simulink model "test_com_AdaptiveTireModel"  (R2017a)
settings: Solver=FixedStepDiscrete  StartTime=450  StopTime=650  RelTol=1e-3
undefined symbols (not defined in the file or in its folder): AxleFrontX, AxleRearX, GearRatio, TireRDyn, TrackAngleFront, TrackWidthFront, TrackWidthRear
settings Model: DataDictionary=controller_dict.sldd  Creator=rieth  LastModifiedBy=rieth
settings DataIOCC: ExternalInput=VD_SteeringAngle_Value, VD_V2O_SpeedLongitudinal, VD_V2O_SpeedLateral, PT_Motor_MotorSpeed_FL, PT_Motor_MotorSpeed_FR, PT_Motor_MotorSpeed_RL, PT_Motor_MotorSpeed_RR, VD_Gyro_Front_Accel_X, VD_Gyro_Front_Accel_Y, VD_Gyro_Front_Accel_Z, VD_Gyro_Front_ARate_X, VD_Gyro_Front_ARate_Y, VD_Gyro_Front_ARate_Z, VD_Gyro_Front_Comp_X, VD_Gyro_Front_Comp_Y, VD_Gyro_Front_Comp_Z, VD_Gyro_Front_Temp, VD_Gyro_Rear_Accel_X, VD_Gyro_Rear_Accel_Y, VD_Gyro_Rear_Accel_Z, VD_Gyro_Rear_ARate_X, VD_Gyro_Rear_ARate_Y,VD_Gyro_Rear_ARate_Z, VD_Gyro_Rear_Comp_X, VD_Gyro_Rear_Comp_Y, VD_Gyro_Rear_Comp_Z, VD_Gyro_Rear_Temp, PT_TorqueCurrent_FL, PT_TorqueCurrent_FR, PT_TorqueCurrent_RL, PT_TorqueCurrent_RR,VD_Suspension_Hall_FL,VD_Suspension_Hall_FR,VD_Suspension_Hall_RL,VD_Suspension_Hall_RR  LoadExternalInput=on
settings OptimizationCC: UseDivisionForNetSlopeComputation=on

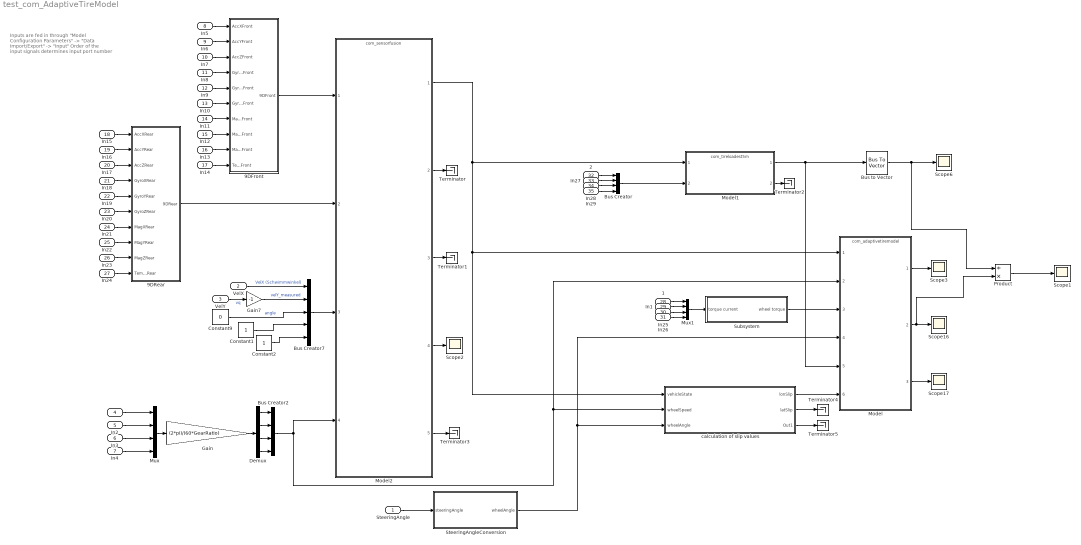
== system test_com_AdaptiveTireModel ==
  note: Inputs are fed in through "Model Configuration Parameters" ->
      | "Data Import/Export" -> "Input"
      | Order of the input signals determines input port number
  SteeringAngle : Inport  OutDataTypeStr=single  Interpolate=off
  VelX : Inport  Port=2  OutDataTypeStr=single
  VelY : Inport  Port=3  OutDataTypeStr=single
  " " : Inport  Port=4  OutDataTypeStr=single
  In2 : Inport  Port=5  OutDataTypeStr=single
  In3 : Inport  Port=6  OutDataTypeStr=single
  In4 : Inport  Port=7  OutDataTypeStr=single
  In5 : Inport  Port=8
  In6 : Inport  Port=9
  In7 : Inport  Port=10
  In8 : Inport  Port=11
  In9 : Inport  Port=12
  In10 : Inport  Port=13
  In11 : Inport  Port=14
  In12 : Inport  Port=15
  In13 : Inport  Port=16
  In14 : Inport  Port=17
  In15 : Inport  Port=18
  In16 : Inport  Port=19
  In17 : Inport  Port=20
  In18 : Inport  Port=21
  In19 : Inport  Port=22
  In20 : Inport  Port=23
  In21 : Inport  Port=24
  In22 : Inport  Port=25
  In23 : Inport  Port=26
  In24 : Inport  Port=27
  " 1" : Inport  Port=28  OutDataTypeStr=single
  In1 : Inport  Port=29  OutDataTypeStr=single
  In25 : Inport  Port=30  OutDataTypeStr=single
  In26 : Inport  Port=31  OutDataTypeStr=single
  " 2" : Inport  Port=32  OutDataTypeStr=single
  In27 : Inport  Port=33  OutDataTypeStr=single
  In28 : Inport  Port=34  OutDataTypeStr=single
  In29 : Inport  Port=35  OutDataTypeStr=single
  9DFront : Subsystem
  9DRear : Subsystem
  Bus Creator : BusCreator  Inputs=4  OutDataTypeStr=Bus: control_LinPot
  Bus Creator2 : BusCreator  Inputs=4  OutDataTypeStr=Bus: control_WheelSpeed
      settings: InheritFromInputs=off
  Bus Creator7 : BusCreator  Inputs=5  OutDataTypeStr=Bus: control_velocity
      settings: InheritFromInputs=off
  Bus to Vector : BusToVector
  Constant1 : Constant  OutDataTypeStr=Inherit: Inherit via back propagation
  Constant2 : Constant  OutDataTypeStr=Inherit: Inherit via back propagation
  Constant9 : Constant  Value=0  OutDataTypeStr=Inherit: Inherit via back propagation
  Demux : Demux
  Gain : Gain  Gain=(2*pi)/(60*GearRatio)
  Gain7 : Gain  Gain=-1
  Model : ModelReference  ModelNameDialog=com_adaptivetiremodel.slx  SimulationMode=Normal  ModelReferenceVersion=1.201
  Model1 : ModelReference  ModelNameDialog=com_tireloadest5m.slx  SimulationMode=Normal  ModelReferenceVersion=1.119
  Model2 : ModelReference  ModelNameDialog=com_sensorfusion.slx  SimulationMode=Normal  ModelReferenceVersion=1.1509
  Mux : Mux
  Mux1 : Mux
  Product : Product  Inputs=/*
  Scope{1..3,6,16..17} (6 alike) : Scope
  SteeringAngleConversion : Subsystem
  Subsystem : Subsystem
  Terminator{,1..5} (6 alike) : Terminator
  calculation of slip values : Subsystem
  wires:
  Model2/1 -> Model1/1, calculation of slip values/1(vehicleState), Model/1
  Model2/2 -> Terminator/1
  Model2/3 -> Terminator1/1
  Model1/1 -> Model/5, Bus to Vector/1
  Model/1 -> Scope3/1
  In23/1 -> 9DRear/9(MagZRear)
  In18/1 -> 9DRear/4(GyroXRear)
  In26/1 -> Mux1/4
  " 1"/1 -> Mux1/1
  Demux/3 -> Bus Creator2/3
  VelY/1 -> Gain7/1  "vq"
  Bus Creator7/1 -> Model2/3
  SteeringAngle/1 -> SteeringAngleConversion/1("steeringAngle ")
  In10/1 -> 9DFront/6(GyroZFront)
  VelX/1 -> Bus Creator7/1  "VelX (Schwimmwinkel)"
  Mux/1 -> Gain/1
  Subsystem/1(wheel torque) -> Model/3
  In1/1 -> Mux1/2
  In20/1 -> 9DRear/6(GyroZRear)
  Model/3 -> Scope17/1
  In16/1 -> 9DRear/2(AccYRear)
  In13/1 -> 9DFront/9(MagZFront)
  In12/1 -> 9DFront/8(MagYFront)
  In24/1 -> 9DRear/10(Temp9DRear)
  " "/1 -> Mux/1
  Demux/2 -> Bus Creator2/2
  Bus Creator2/1 -> Model2/4, Model/2, calculation of slip values/2(wheelSpeed)
  Gain7/1 -> Bus Creator7/2  "velY_measured"
  Constant9/1 -> Bus Creator7/3  "angle"
  Mux1/1 -> Subsystem/1(torque current)
  In15/1 -> 9DRear/1(AccXRear)
  In19/1 -> 9DRear/5(GyroYRear)
  In4/1 -> Mux/4
  In8/1 -> 9DFront/4(GyroXFront)
  In6/1 -> 9DFront/2(AccYFront)
  In2/1 -> Mux/2
  In5/1 -> 9DFront/1(AccXFront)
  In7/1 -> 9DFront/3(AccZFront)
  In14/1 -> 9DFront/10(Temp9DFront)
  Gain/1 -> Demux/1
  In17/1 -> 9DRear/3(AccZRear)
  In21/1 -> 9DRear/7(MagXRear)
  Demux/4 -> Bus Creator2/4
  In3/1 -> Mux/3
  In11/1 -> 9DFront/7(MagXFront)
  In25/1 -> Mux1/3
  In9/1 -> 9DFront/5(GyroYFront)
  Demux/1 -> Bus Creator2/1
  9DFront/1(9DFront) -> Model2/1
  Model/2 -> Product/2, Scope16/1
  9DRear/1(9DRear) -> Model2/2
  In22/1 -> 9DRear/8(MagYRear)
  Model2/5 -> Terminator3/1
  Model2/4 -> Scope2/1
  In28/1 -> Bus Creator/3
  In27/1 -> Bus Creator/2
  " 2"/1 -> Bus Creator/1
  In29/1 -> Bus Creator/4
  Bus Creator/1 -> Model1/2
  Model1/2 -> Terminator2/1
  Constant1/1 -> Bus Creator7/4
  Constant2/1 -> Bus Creator7/5
  Bus to Vector/1 -> Product/1, Scope6/1
  Product/1 -> Scope1/1
  calculation of slip values/2(latSlip) -> Terminator4/1
  calculation of slip values/1(lonSlip) -> Model/6
  calculation of slip values/3(Out1) -> Terminator5/1
  SteeringAngleConversion/1(wheelAngle) -> Model/4, calculation of slip values/3(wheelAngle)

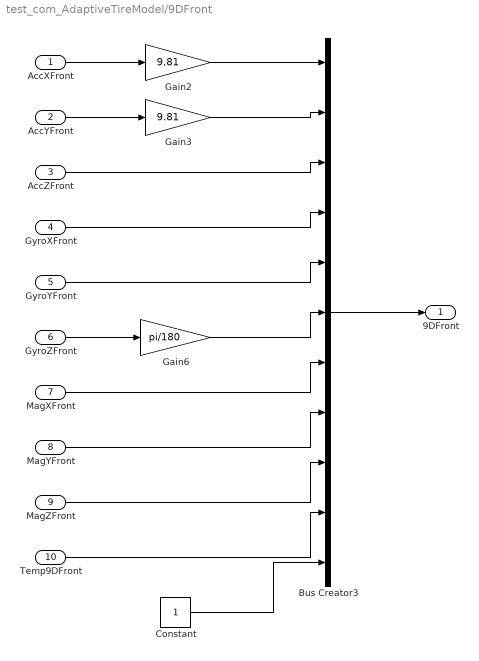
== system test_com_AdaptiveTireModel/9DFront ==
  AccXFront : Inport
  AccYFront : Inport  Port=2
  AccZFront : Inport  Port=3
  GyroXFront : Inport  Port=4
  GyroYFront : Inport  Port=5
  GyroZFront : Inport  Port=6
  MagXFront : Inport  Port=7
  MagYFront : Inport  Port=8
  MagZFront : Inport  Port=9
  Temp9DFront : Inport  Port=10
  Bus Creator3 : BusCreator  Inputs=11  OutDataTypeStr=Bus: control_9D_Full_float
      settings: InheritFromInputs=off
  Constant : Constant  OutDataTypeStr=Inherit: Inherit via back propagation
  Gain2 : Gain  Gain=9.81
  Gain3 : Gain  Gain=9.81
  Gain6 : Gain  Gain=pi/180
  9DFront : Outport
  wires:
  AccXFront/1 -> Gain2/1
  Temp9DFront/1 -> Bus Creator3/10
  GyroZFront/1 -> Gain6/1
  AccZFront/1 -> Bus Creator3/3
  AccYFront/1 -> Gain3/1
  GyroYFront/1 -> Bus Creator3/5
  MagZFront/1 -> Bus Creator3/9
  Gain2/1 -> Bus Creator3/1
  Bus Creator3/1 -> 9DFront/1
  MagYFront/1 -> Bus Creator3/8
  MagXFront/1 -> Bus Creator3/7
  Gain6/1 -> Bus Creator3/6
  GyroXFront/1 -> Bus Creator3/4
  Gain3/1 -> Bus Creator3/2
  Constant/1 -> Bus Creator3/11

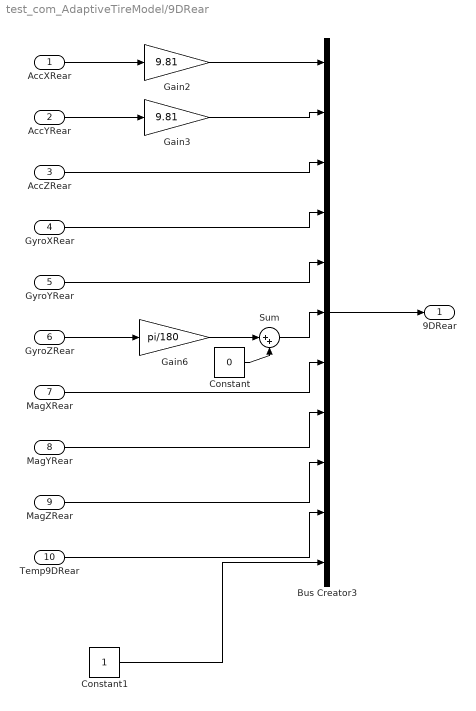
== system test_com_AdaptiveTireModel/9DRear ==
  AccXRear : Inport
  AccYRear : Inport  Port=2
  AccZRear : Inport  Port=3
  GyroXRear : Inport  Port=4
  GyroYRear : Inport  Port=5
  GyroZRear : Inport  Port=6
  MagXRear : Inport  Port=7
  MagYRear : Inport  Port=8
  MagZRear : Inport  Port=9
  Temp9DRear : Inport  Port=10
  Bus Creator3 : BusCreator  Inputs=11  OutDataTypeStr=Bus: control_9D_Full_float
      settings: InheritFromInputs=off
  Constant : Constant  Value=0  OutDataTypeStr=single
  Constant1 : Constant  OutDataTypeStr=Inherit: Inherit via back propagation
  Gain2 : Gain  Gain=9.81
  Gain3 : Gain  Gain=9.81
  Gain6 : Gain  Gain=pi/180
  Sum : Sum  Inputs=|++
  9DRear : Outport
  wires:
  GyroXRear/1 -> Bus Creator3/4
  Gain6/1 -> Sum/1
  MagXRear/1 -> Bus Creator3/7
  MagYRear/1 -> Bus Creator3/8
  Bus Creator3/1 -> 9DRear/1
  Gain3/1 -> Bus Creator3/2
  Gain2/1 -> Bus Creator3/1
  MagZRear/1 -> Bus Creator3/9
  GyroYRear/1 -> Bus Creator3/5
  AccYRear/1 -> Gain3/1
  AccZRear/1 -> Bus Creator3/3
  GyroZRear/1 -> Gain6/1
  Temp9DRear/1 -> Bus Creator3/10
  AccXRear/1 -> Gain2/1
  Sum/1 -> Bus Creator3/6
  Constant/1 -> Sum/2
  Constant1/1 -> Bus Creator3/11

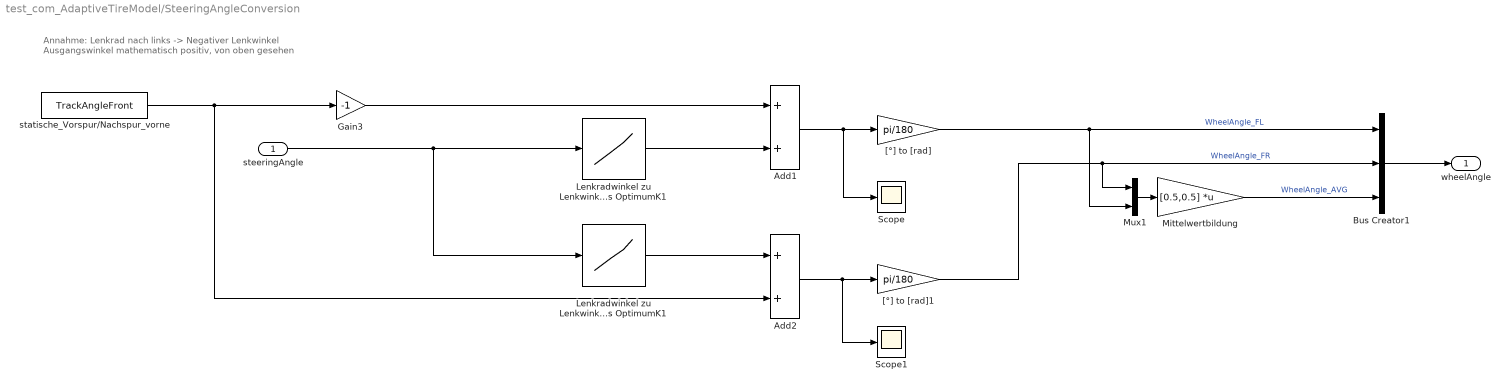
== system test_com_AdaptiveTireModel/SteeringAngleConversion ==
  note: Annahme: Lenkrad nach links -> Negativer Lenkwinkel
      | Ausgangswinkel mathematisch positiv, von oben gesehen
  "steeringAngle " : Inport  Unit=deg
  Add1 : Sum
  Add2 : Sum
  Bus Creator1 : BusCreator  Inputs=3  OutDataTypeStr=Bus: control_WheelAngle
  Gain3 : Gain  Gain=-1
  Lenkradwinkel zu Lenkwinkel_vl aus OptimumK1 : Lookup_n-D  NumberOfTableDimensions=1  BreakpointsForDimension1=|  Table=|  InternalRulePriority=Speed  RndMeth=Simplest  InputSameDT=on
      BreakpointsForDimension1=|
      | [-110
      | -99
      | -88
      | -77
      | -66
      | -55
      | -44
      | -33
      | -22
      | -11
      | 0
      | 11
      | 22
      | 33
      | 44
      | 55
      | 66
      | 77
      | 88
      | 99
      | 110]
      Table=|
      | [-31.406
      | -27.9
      | -24.526
      | -21.258
      | -18.075
      | -14.961
      | -11.902
      | -8.886
      | -5.903
      | -2.944
      | 0
      | 2.937
      | 5.874
      | 8.819
      | 11.78
      | 14.765
      | 17.781
      | 20.838
      | 23.945
      | 27.115
      | 30.358]
  Lenkradwinkel zu Lenkwinkel_vr aus OptimumK1 : Lookup_n-D  NumberOfTableDimensions=1  BreakpointsForDimension1=|  Table=|  InternalRulePriority=Speed  RndMeth=Simplest  InputSameDT=on
      BreakpointsForDimension1=|
      | [-110
      | -99
      | -88
      | -77
      | -66
      | -55
      | -44
      | -33
      | -22
      | -11
      | 0
      | 11
      | 22
      | 33
      | 44
      | 55
      | 66
      | 77
      | 88
      | 99
      | 110]
      Table=|
      | [-30.358
      | -27.115
      | -23.945
      | -20.838
      | -17.781
      | -14.765
      | -11.78
      | -8.819
      | -5.874
      | -2.937
      | 0
      | 2.944
      | 5.903
      | 8.886
      | 11.902
      | 14.961
      | 18.075
      | 21.258
      | 24.526
      | 27.9
      | 31.406]
  Mittelwertbildung : Gain  Gain=[0.5,0.5]  Multiplication=Matrix(K*u)
  Mux1 : Mux  Inputs=2
  Scope : Scope
  Scope1 : Scope
  "[°] to [rad]" : Gain  Gain=pi/180
  "[°] to [rad]1" : Gain  Gain=pi/180
  statische_Vorspur/Nachspur_vorne : Constant  Value=TrackAngleFront
  wheelAngle : Outport
  wires:
  Add2/1 -> Scope1/1, "[°] to [rad]1"/1
  statische_Vorspur/Nachspur_vorne/1 -> Add2/2, Gain3/1
  Lenkradwinkel zu Lenkwinkel_vl aus OptimumK1/1 -> Add1/2
  Lenkradwinkel zu Lenkwinkel_vr aus OptimumK1/1 -> Add2/1
  Gain3/1 -> Add1/1
  "steeringAngle "/1 -> Lenkradwinkel zu Lenkwinkel_vr aus OptimumK1/1, Lenkradwinkel zu Lenkwinkel_vl aus OptimumK1/1
  "[°] to [rad]"/1 -> Bus Creator1/1, Mux1/2  "WheelAngle_FL"
  Add1/1 -> "[°] to [rad]"/1, Scope/1
  "[°] to [rad]1"/1 -> Bus Creator1/2, Mux1/1  "WheelAngle_FR"
  Bus Creator1/1 -> wheelAngle/1
  Mux1/1 -> Mittelwertbildung/1
  Mittelwertbildung/1 -> Bus Creator1/3  "WheelAngle_AVG"

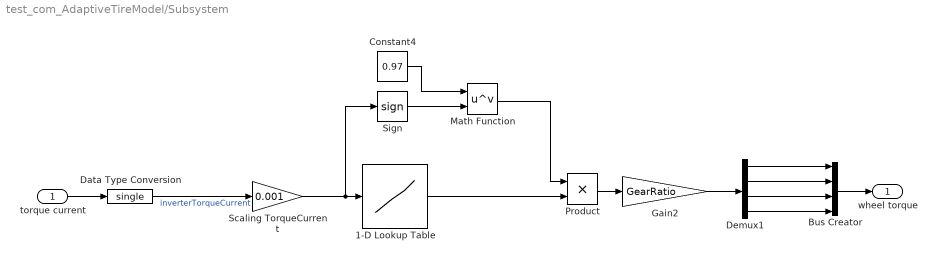
== system test_com_AdaptiveTireModel/Subsystem ==
  torque current : Inport
  1-D Lookup Table : Lookup_n-D  NumberOfTableDimensions=1  BreakpointsForDimension1=single([-98.31700100000001 -91.605003 -83.987999 -76.350998 -68.718002 -61.085999 -53.451 -45.814999 -38.173 -30.547001 -27.493999 -24.450001 -21.4 -18.35 -15.3 -12.26 -9.2110004 -6.1700001 -3.142 0 3.142 6.1700001 9.2110004 12.26 15.3 18.35 21.4 24.450001 27.493999 30.547001 38.173 45.814999 53.451 61.085999 68.718002 76.350998 83.987999 91.605003 98.31700100000001])  Table=single([-27.7 -26.7 -25.5 -24.1 -22.4 -20.5 -18.5 -16.2 -13.8 -11.2 -10.1 -9 -7.8 -6.7 -5.5 -4.4 -3.3 -2.1 -0.9 0 0.9 2.1 3.3 4.4 5.5 6.7 7.8 9 10.1 11.2 13.8 16.2 18.5 20.5 22.4 24.1 25.5 26.7 27.7])  InternalRulePriority=Speed  RndMeth=Simplest  InputSameDT=on
  Bus Creator : BusCreator  Inputs=4  OutDataTypeStr=Bus: control_WheelTorque
      settings: InheritFromInputs=off
  Constant4 : Constant  Value=0.97  OutDataTypeStr=Inherit: Inherit via back propagation
  Data Type Conversion : DataTypeConversion  OutDataTypeStr=single
  Demux1 : Demux
  Gain2 : Gain  Gain=GearRatio
  Math Function : Math  Operator=pow  OutputSignalType=real  SaturateOnIntegerOverflow=on
  Product : Product
  Scaling TorqueCurrent : Gain  Gain=0.001
  Sign : Signum
  wheel torque : Outport  OutDataTypeStr=Bus: control_WheelTorque
  wires:
  Bus Creator/1 -> wheel torque/1
  Gain2/1 -> Demux1/1
  Demux1/4 -> Bus Creator/4
  Demux1/1 -> Bus Creator/1
  Demux1/2 -> Bus Creator/2
  Demux1/3 -> Bus Creator/3
  torque current/1 -> Data Type Conversion/1
  Product/1 -> Gain2/1
  Math Function/1 -> Product/1
  1-D Lookup Table/1 -> Product/2
  Constant4/1 -> Math Function/1
  Data Type Conversion/1 -> Scaling TorqueCurrent/1  "inverterTorqueCurrent"
  Scaling TorqueCurrent/1 -> Sign/1, 1-D Lookup Table/1
  Sign/1 -> Math Function/2

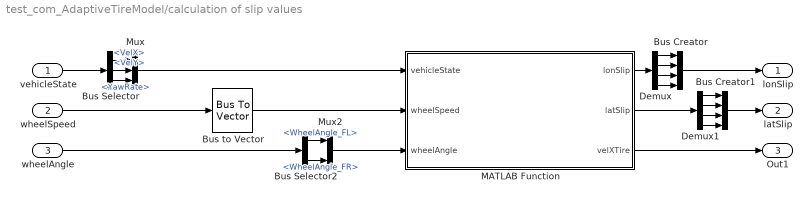
== system test_com_AdaptiveTireModel/calculation of slip values ==
  vehicleState : Inport  OutDataTypeStr=Bus: control_VehicleStateRB
  wheelSpeed : Inport  Port=2  OutDataTypeStr=Bus: control_WheelSpeed
  wheelAngle : Inport  Port=3  OutDataTypeStr=Bus: control_WheelAngle
  Bus Creator : BusCreator  Inputs=4  OutDataTypeStr=Bus: control_LonSlip
      settings: InheritFromInputs=off
  Bus Creator1 : BusCreator  Inputs=4  OutDataTypeStr=Bus: control_LatSlip
      settings: InheritFromInputs=off
  Bus Selector : BusSelector  OutputSignals=VelX,VelY,YawRate
  Bus Selector2 : BusSelector  OutputSignals=WheelAngle_FL,WheelAngle_FR
  Bus to Vector : BusToVector
  Demux : Demux
  Demux1 : Demux
  MATLAB Function : MATLAB Function  TreatAsAtomicUnit=on
  Mux : Mux  Inputs=3
  Mux2 : Mux  Inputs=2
  lonSlip : Outport
  latSlip : Outport  Port=2
  Out1 : Outport  Port=3
  wires:
  Bus Selector/3 -> Mux/3  "<YawRate>"
  Mux/1 -> MATLAB Function/1(vehicleState)
  vehicleState/1 -> Bus Selector/1
  Bus Selector/2 -> Mux/2  "<VelY>"
  Demux1/4 -> Bus Creator1/4
  wheelSpeed/1 -> Bus to Vector/1
  Bus to Vector/1 -> MATLAB Function/2(wheelSpeed)
  Bus Selector/1 -> Mux/1  "<VelX>"
  Bus Creator1/1 -> latSlip/1
  MATLAB Function/1(lonSlip) -> Demux/1
  wheelAngle/1 -> Bus Selector2/1
  Mux2/1 -> MATLAB Function/3(wheelAngle)
  Demux/4 -> Bus Creator/4
  Demux/1 -> Bus Creator/1
  Bus Creator/1 -> lonSlip/1
  Bus Selector2/1 -> Mux2/1  "<WheelAngle_FL>"
  Demux1/3 -> Bus Creator1/3
  Demux/2 -> Bus Creator/2
  MATLAB Function/2(latSlip) -> Demux1/1
  Demux1/1 -> Bus Creator1/1
  Demux1/2 -> Bus Creator1/2
  Bus Selector2/2 -> Mux2/2  "<WheelAngle_FR>"
  Demux/3 -> Bus Creator/3
  MATLAB Function/3(velXTire) -> Out1/1

== matlab function test_com_AdaptiveTireModel/calculation of slip values/MATLAB Function ==
  data: vehicleState input single; wheelSpeed input single; lonSlip output single size=[1,4]; wheelAngle input single; latSlip output single size=[1,4]; TireRDyn parameter; AxleFrontX parameter; AxleRearX parameter; TrackWidthFront parameter; TrackWidthRear parameter; velXTire output
function [lonSlip, latSlip, velXTire] =  MATLAB_Function( vehicleState, wheelSpeed, wheelAngle, TireRDyn, AxleFrontX, AxleRearX, TrackWidthFront, TrackWidthRear)
%#codegen
velRelX=single([0,0,0,0]);
% v_r = omega*r - v_x
% wheelAngleLeft/Right: positiv bei Rechtskurve
% gierrate positiv bei rechtskurve
velX=single([0,0,0,0]);
velY=single([0,0,0,0]);

vel = single([0,0]);
vel(1) = vehicleState(1);
vel(2) = vehicleState(2);
yaw = vehicleState(3);

velX(1) = cos(wheelAngle(1))*(vel(1)+yaw*TrackWidthFront/2) + sin(wheelAngle(1))*(vel(2)+yaw*AxleFrontX);
velX(2) = cos(wheelAngle(2))*(vel(1)-yaw*TrackWidthFront/2) + sin(wheelAngle(2))*(vel(2)+yaw*AxleFrontX);
velX(3) = vel(1)+ yaw*TrackWidthRear/2;
velX(4) = vel(1)- yaw*TrackWidthRear/2;

velY(1) = -sin(wheelAngle(1))*(vel(1)+yaw*TrackWidthFront/2) + cos(wheelAngle(1))*(vel(2)+yaw*AxleFrontX);
velY(2) = -sin(wheelAngle(2))*(vel(1)-yaw*TrackWidthFront/2) + cos(wheelAngle(2))*(vel(2)+yaw*AxleFrontX);
velY(3) = vel(2)- yaw*AxleRearX;
velY(4) = vel(2)- yaw*AxleRearX;

velRelX(1) = wheelSpeed(1)*TireRDyn - velX(1);
velRelX(2) = wheelSpeed(2)*TireRDyn - velX(2);
velRelX(3) = wheelSpeed(3)*TireRDyn - velX(3);
velRelX(4) = wheelSpeed(4)*TireRDyn - velX(4);
if(velX(1) < 0.1)
    latSlip=single([0,0,0,0]);
    lonSlip = single([0,0,0,0]);
else
    latSlip = velY ./ abs(velX);
    lonSlip = velRelX ./ velX;
end
velXTire = velX;
end
